simulink model "kalman_filter"  (R2021b)
settings: Solver=FixedStepDiscrete  StartTime=0.0  StopTime=10.0  FixedStep=Ts  RelTol=1e-3
InitFcn:
  | init;
values from neighbouring files (symbols this model uses):
  R = 1e-4    (= 0.0001)    [init.m]
  sysd = c2d(sys, Ts, 'zoh')    [init.m]
  Ts = 0.001    [init.m]
  x0 = zeros(3, 1)    [init.m]
undefined symbols (not defined in the file or in its folder): Discrete, Time
libraries: ctrlSharedLib x1
settings Model: Creator=upattacini  LastModifiedBy=upattacini
settings DataIOCC: SaveOutput=off  DSMLogging=off  SaveTime=off  ReturnWorkspaceOutputs=off
settings OptimizationCC: DefaultParameterBehavior=Inlined  DefaultUnderspecifiedDataType=single  StrengthReduction=on  PassReuseOutputArgsAs=Individual arguments  ZeroExternalMemoryAtStartup=off  ZeroInternalMemoryAtStartup=off  OptimizeBlockOrder=speed  OptimizationPriority=Speed  OptimizationCustomize=off  MultiThreadedLoops=on  EfficientTunableParamExpr=on
settings DebuggingCC: ParameterTunabilityLossMsg=error
settings HardwareCC: ProdBitPerPointer=32  ProdBitPerSizeT=32  ProdBitPerPtrDiffT=32  ProdLargestAtomicInteger=Long  ProdLargestAtomicFloat=Double  ProdWordSize=32  ProdHWDeviceType=ARM Compatible->ARM Cortex-M
settings SFSimCC: MATLABDynamicMemAlloc=off
settings RTWCC: Description=Embedded Coder  SystemTargetFile=ert.tlc  GenCodeOnly=on  PackageGeneratedCodeAndArtifacts=on  PackageName=kalman_filter  TemplateMakefile=ert_default_tmf  TargetLang=C++
settings CodeAppCC: ForceParamTrailComments=on  IgnoreCustomStorageClasses=off  OperatorAnnotations=on  SimulinkDataObjDesc=on  SFDataObjDesc=on  InsertBlockDesc=on
settings ERTTargetCC: TargetLangStandard=C++11 (ISO)  GenerateSampleERTMain=on  CodeInterfacePackaging=C++ class  InlinedParameterPlacement=NonHierarchical  RootIOFormat=Structure reference  ERTCustomFileTemplate=example_file_process.tlc

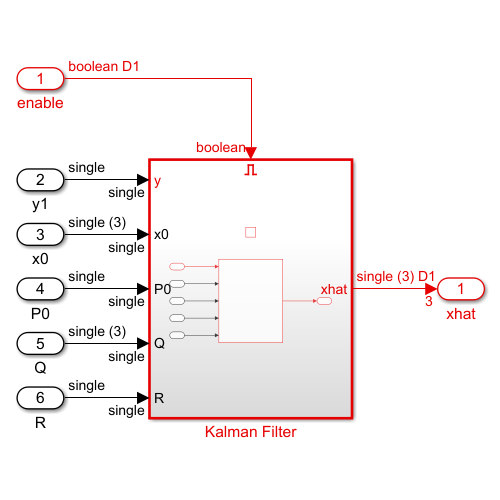
[thumbnail: Simulink's stored preview of the top-level diagram]
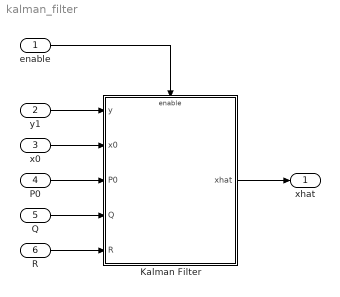
== system kalman_filter ==
  enable : Inport  OutDataTypeStr=boolean  PortDimensions=1  SampleTime=Ts
  y1 : Inport  Port=2  OutDataTypeStr=single  PortDimensions=1  SampleTime=Ts
  x0 : Inport  Port=3  OutDataTypeStr=single  PortDimensions=3  SampleTime=Ts
  P0 : Inport  Port=4  OutDataTypeStr=single  PortDimensions=1  SampleTime=Ts
  Q : Inport  Port=5  OutDataTypeStr=single  PortDimensions=3  SampleTime=Ts
  R : Inport  Port=6  OutDataTypeStr=single  PortDimensions=1  SampleTime=Ts
  Kalman Filter : Subsystem  TreatAsAtomicUnit=on
  xhat : Outport
  wires:
  Kalman Filter/1(xhat) -> xhat/1
  enable/1 -> Kalman Filter/Enable
  y1/1 -> Kalman Filter/1(y)
  x0/1 -> Kalman Filter/2(x0)
  P0/1 -> Kalman Filter/3(P0)
  Q/1 -> Kalman Filter/4(Q)
  R/1 -> Kalman Filter/5(R)

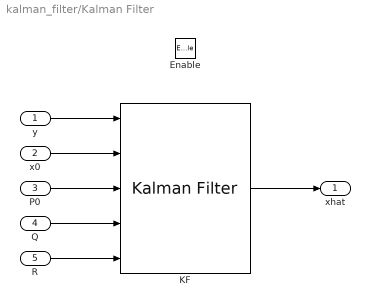
== system kalman_filter/Kalman Filter ==
  y : Inport  OutDataTypeStr=single
  x0 : Inport  Port=2  OutDataTypeStr=single
  P0 : Inport  Port=3  OutDataTypeStr=single
  Q : Inport  Port=4  OutDataTypeStr=single
  R : Inport  Port=5  OutDataTypeStr=single
  Enable : EnablePort  StatesWhenEnabling=reset
  KF : ctrlSharedLib/Kalman Filter  TimeDomain=Discrete-Time  UseCurrentEstimator=on  ModelSource=Individual A, B, C, D matrices  ModelSourceVariable=ss(0.95,1,1,0,1)  A=sysd.A  B=1  C=sysd.C  D=0  NumberOfStates=3  NumberOfInputs=0  NumberOfOutputs=1  InitialEstimateSource=Input port  X0=x0  P0=P0  UseK=off  UseGH=off  NumberOfProcessNoiseInputs=1  G=1  TimeInvariantG=on  H=0  TimeInvariantH=on  Q=Q  TimeInvariantQ=off  R=R  TimeInvariantR=off  N=0  TimeInvariantN=on  AddInputPort=off  AddEnablePort=off  OutputEstimatedY=off  OutputP=off  Ts=-1
  xhat : Outport
  wires:
  KF/1 -> xhat/1
  y/1 -> KF/1
  x0/1 -> KF/2
  P0/1 -> KF/3
  Q/1 -> KF/4
  R/1 -> KF/5
